simulink model "Tank_Modell_Student"  (R2020b)
settings: Solver=ode45  StartTime=0.0  StopTime=1500  RelTol=1e-3
undefined symbols (not defined in the file or in its folder): parInit, parSys
libraries: simulink x1
settings Model: Creator=Wolfgang Kemmetmüller  LastModifiedBy=Armin Wessel
settings DataIOCC: LimitDataPoints=on  SaveFormat=Array  ReturnWorkspaceOutputs=off
settings OptimizationCC: BlockReduction=off  BooleanDataType=off  LifeSpan=inf
settings DebuggingCC: SaveWithParameterizedLinksMsg=none  UnderspecifiedInitializationDetection=Classic  MergeDetectMultiDrivingBlocksExec=none  SignalResolutionControl=TryResolveAllWithWarning  SFUnexpectedBacktrackingDiag=warning  SFNoUnconditionalDefaultTransitionDiag=warning  SFExecutionAtInitializationDiag=none  ArithmeticOperatorsInVariantConditions=warning
settings HardwareCC: ProdBitPerPointer=32  ProdBitPerSizeT=32  ProdBitPerPtrDiffT=32  ProdLargestAtomicFloat=None  ProdIntDivRoundTo=Undefined  ProdEndianess=Unspecified  ProdWordSize=32  ProdHWDeviceType=32-bit Generic  TargetUnknown=on
settings ModelReferenceCC: PropagateSignalLabelsOutOfModel=off
settings SFSimCC: SimUseLocalCustomCode=off  CustomCodeUndefinedFunction=UseInterfaceOnly
settings RTWCC: RTWUseLocalCustomCode=off
settings CodeAppCC: StateflowObjectComments=on
settings GRTTargetCC: TargetLangStandard=C89/C90 (ANSI)
settings ConfigComp: CovMetricSettings=dw  CovSaveCumulativeToWorkspaceVar=on  CovSaveSingleToWorkspaceVar=on  CovExternalEMLEnable=off

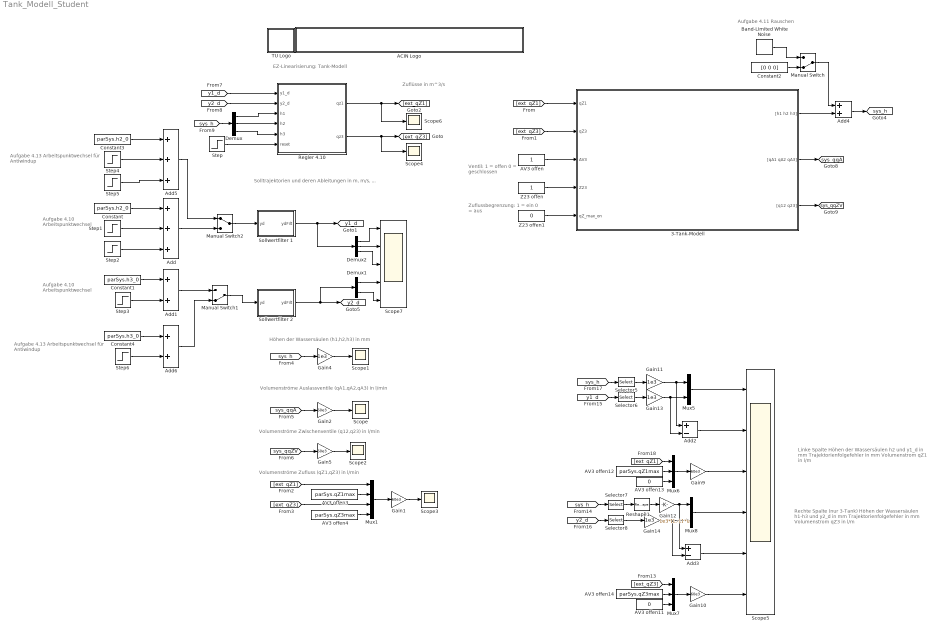
== system Tank_Modell_Student ==
  note: Aufgabe 4.10
      | Arbeitspunktwechsel
  note: Aufgabe 4.11 Rauschen
  note: EZ-Linearisierung: Tank-Modell
  note: Höhen der Wassersäulen (h1,h2,h3) in mm
  note: Volumenströme Auslassventile (qA1,qA2,qA3) in l/min
  note: Volumenströme Zwischenventile (q12,q23) in l/min
  note: Ventil:
      | 1 = offen
      | 0 = geschlossen
  note: Volumenströme Zufluss (qZ1,qZ3) in l/min
  note: Linke Spalte
      | Höhen der Wassersäulen h2 und y1_d in mm
      | Trajektorienfolgefehler in mm
      | Volumenstrom qZ1 in l/m
  note: Zuflussbegrenzung:
      | 1 = ein
      | 0 = aus
  note: Rechte Spalte (nur 3-Tank)
      | Höhen der Wassersäulen h1-h3 und y2_d in mm
      | Trajektorienfolgefehler in mm
      | Volumenstrom qZ3 in l/m
  note: Zuflüsse in m^3/s
  note: Solltrajektorien und deren Ableitungen in m, m/s, ...
  note: Aufgabe 4.10
      | Arbeitspunktwechsel
  note: Aufgabe 4.13
      | Arbeitspunktwechsel für Antiwindup
  note: Aufgabe 4.13
      | Arbeitspunktwechsel für Antiwindup
  3-Tank-Modell : Subsystem
      mask init:
      | S = get_param(gcb,'UserData');
      mask Display:
      | image(S.pic);
      | port_label('input', 1, 'qZ1');
      | port_label('input', 2, 'qZ3');
      | port_label('input', 3, 'AV3');
      | port_label('input', 4, 'Z23');
      | port_label('input', 5, 'q_max_on');
      | port_label('output', 1, '[h1 h2 h3]');
      | port_label('output', 2, '[qA1 qA2 qA3]');
      | port_label('output', 3, '[q12 q23]');
  ACIN Logo : Subsystem
      mask init:
      | s = get_param(gcb,'UserData');
      mask Display:
      | image(s.logo,[0 0 439 45]);
      | %axis image
  AV3 offen : Constant
  AV3 offen11 : Constant  Value=0
  AV3 offen12 : Constant  Value=parSys.qZ1max  SampleTime=parSys.Ta
  AV3 offen13 : Constant  Value=0
  AV3 offen14 : Constant  Value=parSys.qZ3max  SampleTime=parSys.Ta
  AV3 offen3 : Constant  Value=parSys.qZ1max  SampleTime=parSys.Ta
  AV3 offen4 : Constant  Value=parSys.qZ3max  SampleTime=parSys.Ta
  Add : Sum  Inputs=+++
  Add1 : Sum
  Add2 : Sum  Inputs=+-
  Add3 : Sum  Inputs=+-
  Add4 : Sum
  Add5 : Sum  Inputs=+++
  Add6 : Sum
  Band-Limited White Noise : simulink/Sources/Band-Limited White Noise  Cov=[0.05e-3*0.05e-3, 0.05e-3*0.05e-3, 0.05e-3*0.05e-3]  Ts=0.1  seed=[23341]
  Constant : Constant  Value=parSys.h2_0
  Constant1 : Constant  Value=parSys.h3_0
  Constant2 : Constant  Value=[0 0 0]
  Constant3 : Constant  Value=parSys.h2_0
  Constant4 : Constant  Value=parSys.h3_0
  Demux : Demux  Outputs=3
  Demux1 : Demux  Outputs=2
  Demux2 : Demux  Outputs=3
  Gain{1..2,5,9..10} (5 alike) : Gain  Gain=60e3
  Gain{4,11,13..14} (4 alike) : Gain  Gain=1e3
  Gain12 : Gain  Gain=1e3*[1,-1]  Multiplication=Matrix(K*u)
  Manual Switch : ManualSwitch  CurrentSetting=0
  Manual Switch1 : ManualSwitch  CurrentSetting=0
  Manual Switch2 : ManualSwitch
  Mux1 : Mux
  Mux5 : Mux  Inputs=2
  Mux6 : Mux  Inputs=3
  Mux7 : Mux  Inputs=3
  Mux8 : Mux  Inputs=2
  Regler 4.10 : MATLAB Function  TreatAsAtomicUnit=on
  Reshape1 : Reshape  OutputDimensionality=Column vector (2-D)
  Scope{,1..4,6} (6 alike) : Scope
  Scope5 : Scope  NumInputPorts=6
  Scope7 : Scope  NumInputPorts=5
  Selector5 : Selector  InputPortWidth=3  IndexOptions=Index vector (dialog)  Indices=[2]  OutputSizes=1
  Selector6 : Selector  InputPortWidth=3  IndexOptions=Index vector (dialog)  Indices=[1]  OutputSizes=1
  Selector7 : Selector  InputPortWidth=3  IndexOptions=Index vector (dialog)  Indices=[1 3]  OutputSizes=1
  Selector8 : Selector  InputPortWidth=2  IndexOptions=Index vector (dialog)  Indices=[1]  OutputSizes=1
  Sollwertfilter 1 : MATLAB Function  TreatAsAtomicUnit=on
  Sollwertfilter 2 : MATLAB Function  TreatAsAtomicUnit=on
  Step : Step  Before=1  After=0  SampleTime=0
  Step1 : Step  Time=0  After=0.1  SampleTime=0
  Step2 : Step  Time=600  After=-0.1  SampleTime=0
  Step3 : Step  Time=300  After=-0.05  SampleTime=0
  Step4 : Step  Time=0  After=0.28  SampleTime=0
  Step5 : Step  Time=600  After=-0.28  SampleTime=0
  Step6 : Step  Time=300  After=-0.15  SampleTime=0
  TU Logo : Subsystem
      mask init:
      | s = get_param(gcb,'UserData');
      mask Display: image(s.logo,[0 0 45 45]);
  Z23 offen : Constant
  Z23 offen1 : Constant  Value=0
  tag scope: sys_h=global, sys_qqA=global, sys_qqZV=global, y1_d=global, y2_d=global
  wires:
  [sys_qqA] -> Gain2/1
  [sys_qqZV] -> Gain5/1
  [sys_h] -> Gain4/1
  3-Tank-Modell/3("[q12 q23]") -> [sys_qqZV]
  3-Tank-Modell/2("[qA1 qA2 qA3]") -> [sys_qqA]
  AV3 offen/1 -> 3-Tank-Modell/3(AV3)
  Z23 offen/1 -> 3-Tank-Modell/4(Z23)
  [ext_qZ1] -> 3-Tank-Modell/1(qZ1)
  [ext_qZ3] -> 3-Tank-Modell/2(qZ3)
  [ext_qZ1] -> Mux1/1
  [ext_qZ3] -> Mux1/3
  AV3 offen3/1 -> Mux1/2
  AV3 offen4/1 -> Mux1/4
  Gain5/1 -> Scope2/1
  Gain2/1 -> Scope/1
  Gain4/1 -> Scope1/1
  Mux1/1 -> Gain1/1
  Gain1/1 -> Scope3/1
  Sollwertfilter 1/1(ydFilt) -> Demux2/1, [y1_d]
  Z23 offen1/1 -> 3-Tank-Modell/5(qZ_max_on)
  Sollwertfilter 2/1(ydFilt) -> Demux1/1, [y2_d]
  [ext_qZ3] -> Mux7/1
  Selector6/1 -> Gain13/1
  Mux7/1 -> Gain10/1
  AV3 offen11/1 -> Mux7/3
  [sys_h] -> Selector7/1
  AV3 offen14/1 -> Mux7/2
  [ext_qZ1] -> Mux6/1
  Selector7/1 -> Reshape1/1
  Reshape1/1 -> Gain12/1
  [y2_d] -> Selector8/1
  Gain14/1 -> Mux8/2, Add3/2
  [sys_h] -> Selector5/1
  [y1_d] -> Selector6/1
  AV3 offen12/1 -> Mux6/2
  AV3 offen13/1 -> Mux6/3
  Selector8/1 -> Gain14/1
  Gain11/1 -> Add2/1, Mux5/1
  Add3/1 -> Scope5/5
  Mux6/1 -> Gain9/1
  Gain9/1 -> Scope5/3
  Selector5/1 -> Gain11/1
  Mux5/1 -> Scope5/1
  Add2/1 -> Scope5/2
  Gain13/1 -> Add2/2, Mux5/2
  Gain12/1 -> Mux8/1, Add3/1
  Mux8/1 -> Scope5/4
  Gain10/1 -> Scope5/6
  Regler 4.10/1(qz1) -> Scope6/1, [ext_qZ1]
  Regler 4.10/2(qz3) -> Scope4/1, [ext_qZ3]
  [y2_d] -> Regler 4.10/2(y2_d)
  [y1_d] -> Regler 4.10/1(y1_d)
  Demux/1 -> Regler 4.10/3(h1)
  Demux/2 -> Regler 4.10/4(h2)
  Demux/3 -> Regler 4.10/5(h3)
  [sys_h] -> Demux/1
  Step/1 -> Regler 4.10/6(reset)
  Constant/1 -> Add/1
  Constant1/1 -> Add1/1
  Step1/1 -> Add/2
  Step2/1 -> Add/3
  Step3/1 -> Add1/2
  3-Tank-Modell/1("[h1 h2 h3]") -> Add4/2
  Add4/1 -> [sys_h]
  Manual Switch/1 -> Add4/1
  Band-Limited White Noise/1 -> Manual Switch/1
  Constant2/1 -> Manual Switch/2
  Manual Switch1/1 -> Sollwertfilter 2/1(yd)
  Add1/1 -> Manual Switch1/1
  Manual Switch2/1 -> Sollwertfilter 1/1(yd)
  Add/1 -> Manual Switch2/2
  Add5/1 -> Manual Switch2/1
  Step5/1 -> Add5/3
  Constant3/1 -> Add5/1
  Step4/1 -> Add5/2
  Add6/1 -> Manual Switch1/2
  Constant4/1 -> Add6/1
  Step6/1 -> Add6/2
  Demux1/2 -> Scope7/5
  Demux1/1 -> Scope7/4
  Demux2/3 -> Scope7/3
  Demux2/2 -> Scope7/2
  Demux2/1 -> Scope7/1

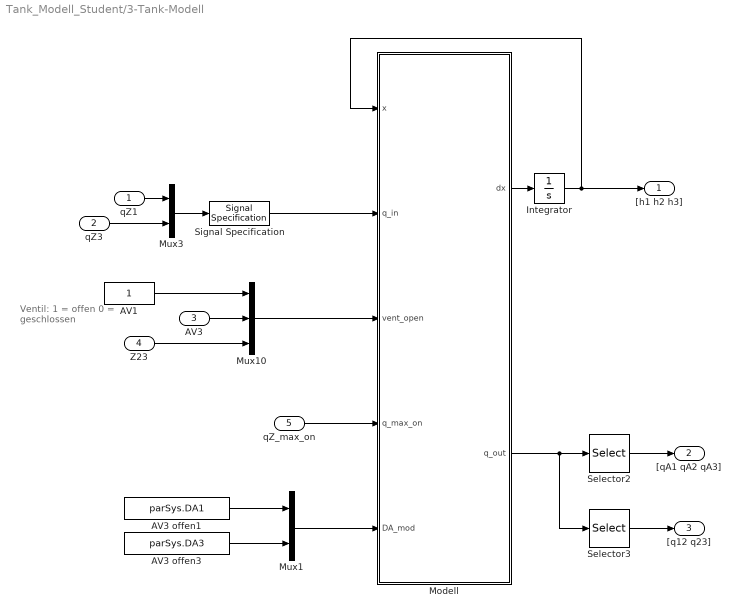
== system Tank_Modell_Student/3-Tank-Modell ==
  note: Ventil:
      | 1 = offen
      | 0 = geschlossen
  qZ1 : Inport
  qZ3 : Inport  Port=2
  AV3 : Inport  Port=3
  Z23 : Inport  Port=4
  qZ_max_on : Inport  Port=5
  AV1 : Constant
  AV3 offen1 : Constant  Value=parSys.DA1
  AV3 offen3 : Constant  Value=parSys.DA3
  Integrator : Integrator  InitialCondition=[parSys.h1_0;parSys.h2_0;parSys.h3_0]
  Modell : MATLAB Function  TreatAsAtomicUnit=on
  Mux1 : Mux  Inputs=2
  Mux10 : Mux  Inputs=3
  Mux3 : Mux  Inputs=2
  Selector2 : Selector  InputPortWidth=5  IndexOptions=Index vector (dialog)  Indices=[1 2 3]  OutputSizes=1
  Selector3 : Selector  InputPortWidth=5  IndexOptions=Index vector (dialog)  Indices=[4 5]  OutputSizes=1
  Signal Specification : SignalSpecification  Dimensions=2
  "[h1 h2 h3]" : Outport  VectorParamsAs1DForOutWhenUnconnected=off
  "[qA1 qA2 qA3]" : Outport  Port=2  VectorParamsAs1DForOutWhenUnconnected=off
  "[q12 q23]" : Outport  Port=3  VectorParamsAs1DForOutWhenUnconnected=off
  wires:
  AV1/1 -> Mux10/1
  qZ1/1 -> Mux3/1
  qZ3/1 -> Mux3/2
  Modell/2(q_out) -> Selector3/1, Selector2/1
  Selector2/1 -> "[qA1 qA2 qA3]"/1
  Selector3/1 -> "[q12 q23]"/1
  Z23/1 -> Mux10/3
  AV3/1 -> Mux10/2
  Mux10/1 -> Modell/3(vent_open)
  Mux3/1 -> Signal Specification/1
  Modell/1(dx) -> Integrator/1
  Integrator/1 -> Modell/1(x), "[h1 h2 h3]"/1
  Mux1/1 -> Modell/5(DA_mod)
  qZ_max_on/1 -> Modell/4(q_max_on)
  AV3 offen1/1 -> Mux1/1
  AV3 offen3/1 -> Mux1/2
  Signal Specification/1 -> Modell/2(q_in)

== system Tank_Modell_Student/ACIN Logo ==

== system Tank_Modell_Student/TU Logo ==

== matlab function Tank_Modell_Student/Sollwertfilter 1 ==
  data: ydFilt output; yd input; parSys parameter
function ydFilt = fcn(yd,parSys)
persistent x
if isempty(x)
    x = parSys.Swy1FilterInit'; 
end

ydFilt = parSys.Cy1Filter*x;
x  = parSys.Ay1Filter*x + parSys.By1Filter*yd;
end

== matlab function Tank_Modell_Student/Regler 4.10 ==
  settings: updateMethod=DISCRETE  sampleTime=parSys.Ta
  data: y1_d input; qz1 output; y2_d input; h1 input; h2 input; h3 input; reset input; qz3 output; parSys parameter; parInit parameter
function [qz1,qz3] = fcn(y1_d,y2_d,h1,h2,h3,reset, parSys, parInit)

persistent errory1;
persistent errory2;

if isempty(errory1)
    errory1 = 0;
    errory2 = 0;
end

if reset == 1
    errory1 = 0;
    errory2 = 0;
end

% Parameter importieren 
Atank       =   parSys.Atank;       % Grundfläche Tank
rho         =   parSys.rho;         % Dichte Wasser
eta         =   parSys.eta;         % Dynamische Viskosität Wasser
g           =   parSys.g;           % Gravitationskonstante
alphaA1     =   parSys.alphaA1;     % Kontraktionskoeffizient AV1
DA1         =   parSys.DA1;         % Durchmesser AV1
alphaA2     =   parSys.alphaA2;     % Kontraktionskoeffizient AV2
A2          =   parSys.A2;          % Querschnittsflaeche AV2
alphaA3     =   parSys.alphaA3;     % Kontraktionskoeffizient AV3
DA3         =   parSys.DA3;         % Durchmesser AV3
alpha120   =   parSys.alpha12_0;   % Kontraktionskoeffizient ZV12
A12         =   parSys.A12;         % Querschnittsflaeche ZV12
Dh12        =   parSys.Dh12;        % hydraulischer Durchmesser
lambdac12   =   parSys.lambdac12;   % kritische Fliesszahl ZV12
alpha230   =   parSys.alpha23_0;   % Kontraktionskoeffizient ZV23
D23         =   parSys.D23;         % Durchmesser ZV23
lambdac23   =   parSys.lambdac23;   % Kritische Fliesszahl ZV23
hmin        =   parSys.hmin;        % Minimale Fuellhoehe
hmax        =   parSys.hmax;        % Maximale Fuellhoehe


    y1a0 = parInit.y1a0;
    y1a1 = parInit.y1a1;
    y2a0 = parInit.y2a0;
    y1aI = parInit.y1aI;
    y2aI = parInit.y2aI;


% y desired werte von Filter
y1d   = y1_d(1);
y1dp  = y1_d(2);
y1dpp = y1_d(3);

y2d   = y2_d(1);
y2dp  = y2_d(2);

%Signum Funktion 
% if h1 - h2 >0  
%     signh1h2 = 1;
% else
%     signh1h2 = -1;
% end
% 
% if h2 - h3 >0  
%     signh2h3 = 1;
% else
%     signh2h3 = -1;
% end
% Umgebung Grenzen für Linearisierung definieren, Geradennäherung aus Maple
deltahmin = 1e-3;
deltah12 = abs(h1 - h2);
deltah23 = abs(h2 - h3); 

if deltah12 < deltahmin 
    dq12dh1 = 0.2381618969e-3 - 0.16030225e-2 * deltah12;
    dq12dh2 = -0.2381618969e-3 + 0.16030225e-2 * deltah12;
else
dq12dh1 = 0.2e1 * alpha120 * Dh12 * rho / eta * g / lambdac12 * (0.1e1 - tanh(0.2e1 * Dh12 * rho / eta * sqrt(0.2e1) * sqrt(g) * sqrt(deltah12) / lambdac12) ^ 2) * A12 + alpha120 * tanh(0.2e1 * Dh12 * rho / eta * sqrt(0.2e1) * sqrt(g) * sqrt(deltah12) / lambdac12) * A12 * sqrt(0.2e1) * sqrt(g) * deltah12 ^ (-0.1e1 / 0.2e1) / 0.2e1;
dq12dh2 = -0.2e1 * alpha120 * Dh12 * rho / eta * g / lambdac12 * (0.1e1 - tanh(0.2e1 * Dh12 * rho / eta * sqrt(0.2e1) * sqrt(g) * sqrt(deltah12) / lambdac12) ^ 2) * A12 - alpha120 * tanh(0.2e1 * Dh12 * rho / eta * sqrt(0.2e1) * sqrt(g) * sqrt(deltah12) / lambdac12) * A12 * sqrt(0.2e1) * sqrt(g) * deltah12 ^ (-0.1e1 / 0.2e1) / 0.2e1;
end

if deltah23 < deltahmin 
    dq23dh3 = -0.5295911873e-3 + 0.88130242e-2 * deltah23;
    dq23dh2 = 0.5295911873e-3 - 0.88130242e-2 * deltah23;

else
dq23dh3 = -alpha230 * D23 ^ 3 * rho / eta * g / lambdac23 * (0.1e1 - tanh(0.2e1 * D23 * rho / eta * sqrt(0.2e1) * sqrt(g) * sqrt(deltah23) / lambdac23) ^ 2) * pi / 0.2e1 - alpha230 * tanh(0.2e1 * D23 * rho / eta * sqrt(0.2e1) * sqrt(g) * sqrt(deltah23) / lambdac23) * D23 ^ 2 * pi * sqrt(0.2e1) * sqrt(g) * deltah23 ^ (-0.1e1 / 0.2e1) / 0.8e1;
dq23dh2 = alpha230 * D23 ^ 3 * rho / eta * g / lambdac23 * (0.1e1 - tanh(0.2e1 * D23 * rho / eta * sqrt(0.2e1) * sqrt(g) * sqrt(deltah23) / lambdac23) ^ 2) * pi / 0.2e1 + alpha230 * tanh(0.2e1 * D23 * rho / eta * sqrt(0.2e1) * sqrt(g) * sqrt(deltah23) / lambdac23) * D23 ^ 2 * pi * sqrt(0.2e1) * sqrt(g) * deltah23 ^ (-0.1e1 / 0.2e1) / 0.8e1;
end


% Gleichungen aus Maple

%Gleichungen
qA1 = alphaA1 * DA1 ^ 2 * pi * sqrt(0.2e1) * sqrt(g) * sqrt(h1) / 0.4e1;
qA2 = alphaA2 * A2 * sqrt(0.2e1) * sqrt(g * h2);
qA3 = 0.7853750000e0 * alphaA3 * DA3 ^ 2 * sqrt(0.2e1) * sqrt(g * h3);
q12 = alpha120 * tanh(0.2e1 * Dh12 * rho / eta * sqrt(0.2e1) * sqrt(g) * sqrt(abs(h1 - h2)) / lambdac12) * A12 * sqrt(0.2e1) * sqrt(g) * sqrt(abs(h1 - h2)) * sign((h1 - h2));
q23 = alpha230 * tanh(0.2e1 * D23 * rho / eta * sqrt(0.2e1) * sqrt(g) * sqrt(abs(h2 - h3)) / lambdac23) * D23 ^ 2 * pi * sqrt(0.2e1) * sqrt(g) * sqrt(abs(h2 - h3)) * sign((h2 - h3)) / 0.4e1;

% Ableitungen nach Parameter
dqA1dh1 = alphaA1 * DA1 ^ 2 * pi * sqrt(0.2e1) * sqrt(g) * h1 ^ (-0.1e1 / 0.2e1) / 0.8e1;
dqA2dh2 = alphaA2 * A2 * sqrt(0.2e1) * sqrt(g) * h2 ^ (-0.1e1 / 0.2e1) / 0.2e1;

% Lie Ableitungen
Lf1h1 = 0.1e1 / Atank * (q12 - q23 - qA2);

%Ausgänge
hh1 = [h2];
hh2 = [h1 - h3];

% Regelgesetz
vWelle = [-y1a1 * (Lf1h1 - y1dp) - y1a0 * (hh1 - y1d) -y2a0 * (hh2 - y2d)]';


    

vWelle = vWelle + [ -y1aI * errory1; -y2aI * errory2];

v = vWelle + ([y1dpp y2dp]');
b = [0.1e1 / Atank ^ 2 * dq12dh1 * (-q12 - qA1) + 0.1e1 / Atank ^ 2 * (dq12dh2 - dq23dh2 - dqA2dh2) * (q12 - q23 - qA2) - 0.1e1 / Atank ^ 2 * dq23dh3 * (q23 - qA3) 0.1e1 / Atank * (-q12 - qA1) - 0.1e1 / Atank * (q23 - qA3)]';
DDInv = [Atank ^ 2 / (dq12dh1 - dq23dh3) -Atank * dq23dh3 / (dq12dh1 - dq23dh3); Atank ^ 2 / (dq12dh1 - dq23dh3) -Atank * dq12dh1 / (dq12dh1 - dq23dh3);];
u = DDInv * (v - b);

%Integral Anteil
if u(1) > parSys.qZ1max || u(1) < 0 || u(2) > parSys.qZ3max  || u(2) < 0 

else
    errory1 = errory1 + parSys.Ta * (hh1 - y1d);
    errory2 = errory2 + parSys.Ta * (hh2 - y2d);
end



if u(1) > parSys.qZ1max & parInit.windup
    qz1 = parSys.qZ1max;
elseif u(1) < 0 & parInit.windup
    qz1 = 0;
else
    qz1 = u(1);
end

if u(2) > parSys.qZ3max & parInit.windup
    qz3 = parSys.qZ3max;
elseif u(2) < 0 & parInit.windup
    qz3 = 0;
else
    qz3 = u(2);
end


end

== matlab function Tank_Modell_Student/Sollwertfilter 2 ==
  data: ydFilt output; yd input; parSys parameter
function ydFilt = fcn(yd,parSys)
persistent x
if isempty(x)
    x = parSys.Swy2FilterInit'; 
end

ydFilt = parSys.Cy2Filter*x;
x  = parSys.Ay2Filter*x + parSys.By2Filter*yd;
end

== matlab function Tank_Modell_Student/3-Tank-Modell/Modell ==
  data: dx output; x input; q_in input; vent_open input; q_max_on input; DA_mod input; q_out output; parSys parameter
function [dx,q_out] = fcn(x,q_in,vent_open,q_max_on,DA_mod,parSys)
%#codegen

[dx,q_out] = Wassertank_mfun(x,q_in,vent_open,q_max_on,DA_mod,parSys);


% Function end
end
